simulink model "serial3_sm_ROS"  (R2022a)
settings: Solver=VariableStepAuto  StartTime=0.0  StopTime=inf  RelTol=1e-3
libraries: robotlib x8
settings Model: Creator=johnc  LastModifiedBy=johnc
settings SolverCC: AlgebraicLoopSolver=TrustRegion
settings DebuggingCC: UnconnectedInputMsg=warning  UnconnectedOutputMsg=warning  UnconnectedLineMsg=warning  SFMachineParentedDataDiag=warning

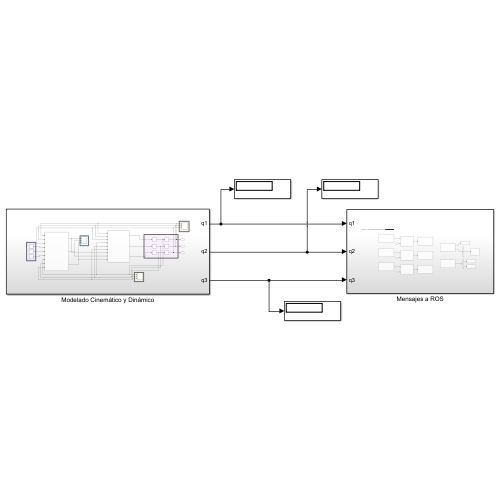
[thumbnail: Simulink's stored preview of the top-level diagram]
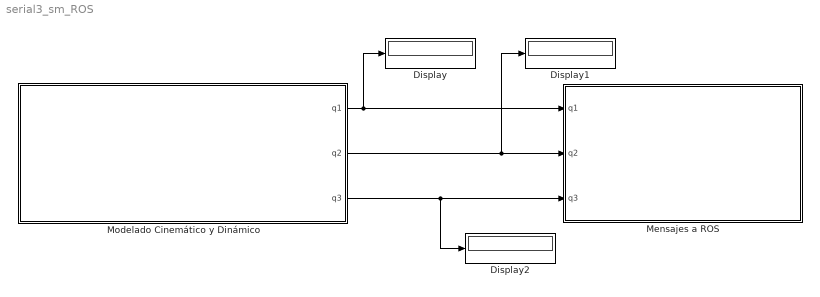
== system serial3_sm_ROS ==
  Display : Display
  Display1 : Display
  Display2 : Display
  Mensajes a ROS : Subsystem
  Modelado Cinemático y Dinámico : Subsystem
  wires:
  Modelado Cinemático y Dinámico/1(q1) -> Display/1, Mensajes a ROS/1(q1)
  Modelado Cinemático y Dinámico/2(q2) -> Display1/1, Mensajes a ROS/2(q2)
  Modelado Cinemático y Dinámico/3(q3) -> Display2/1, Mensajes a ROS/3(q3)

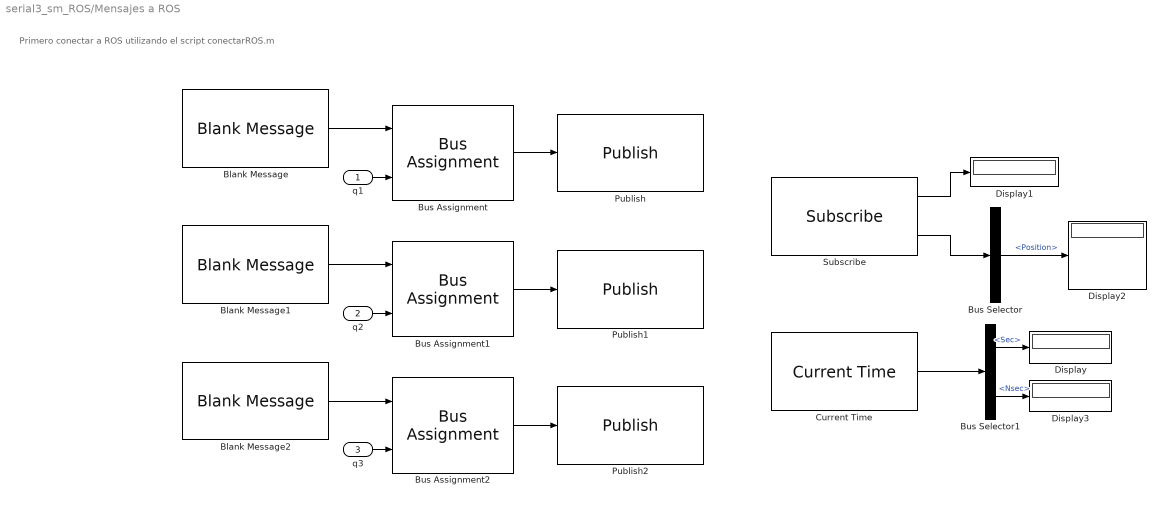
== system serial3_sm_ROS/Mensajes a ROS ==
  note: Primero conectar a ROS utilizando el script conectarROS.m
  q1 : Inport
  q2 : Inport  Port=2
  q3 : Inport  Port=3
  Blank Message : robotlib/Blank Message  messageClass=Message  entityType=std_msgs/Float64  messageType=std_msgs/Float64  SampleTime=inf  legacyBusStruct=off
  Blank Message1 : robotlib/Blank Message  messageClass=Message  entityType=std_msgs/Float64  messageType=std_msgs/Float64  SampleTime=inf  legacyBusStruct=off
  Blank Message2 : robotlib/Blank Message  messageClass=Message  entityType=std_msgs/Float64  messageType=std_msgs/Float64  SampleTime=inf  legacyBusStruct=off
  Bus Assignment : BusAssignment  AssignedSignals=Data
  Bus Assignment1 : BusAssignment  AssignedSignals=Data
  Bus Assignment2 : BusAssignment  AssignedSignals=Data
  Bus Selector : BusSelector  OutputSignals=Position
  Bus Selector1 : BusSelector  OutputSignals=Sec,Nsec
  Current Time : robotlib/Current Time  OutputFormat=bus  SampleTime=-1  ModelName=serial3_modeloROS
      settings: SourceProductBaseCode=RR
  Display{,1..3} (4 alike) : Display
  Publish : robotlib/Publish  topicSource=Select from ROS network  topic=/serial3/joint_e1_position_controller/command  messageType=std_msgs/Float64  legacyBusStruct=off  messageQueueLength=1
  Publish1 : robotlib/Publish  topicSource=Select from ROS network  topic=/serial3/joint_e2_position_controller/command  messageType=std_msgs/Float64  legacyBusStruct=off  messageQueueLength=1
  Publish2 : robotlib/Publish  topicSource=Select from ROS network  topic=/serial3/joint_e3_position_controller/command  messageType=std_msgs/Float64  legacyBusStruct=off  messageQueueLength=1
  Subscribe : robotlib/Subscribe  topicSource=Select from ROS network  topic=/serial3/joint_states  messageType=sensor_msgs/JointState  SampleTime=-1  legacyBusStruct=off  messageQueueLength=1
  wires:
  Blank Message2/1 -> Bus Assignment2/1
  Blank Message/1 -> Bus Assignment/1
  Bus Assignment2/1 -> Publish2/1
  q1/1 -> Bus Assignment/2
  Bus Assignment/1 -> Publish/1
  Blank Message1/1 -> Bus Assignment1/1
  Bus Assignment1/1 -> Publish1/1
  q3/1 -> Bus Assignment2/2
  q2/1 -> Bus Assignment1/2
  Subscribe/2 -> Bus Selector/1
  Subscribe/1 -> Display1/1
  Bus Selector/1 -> Display2/1  "<Position>"
  Current Time/1 -> Bus Selector1/1
  Bus Selector1/1 -> Display/1  "<Sec>"
  Bus Selector1/2 -> Display3/1  "<Nsec>"

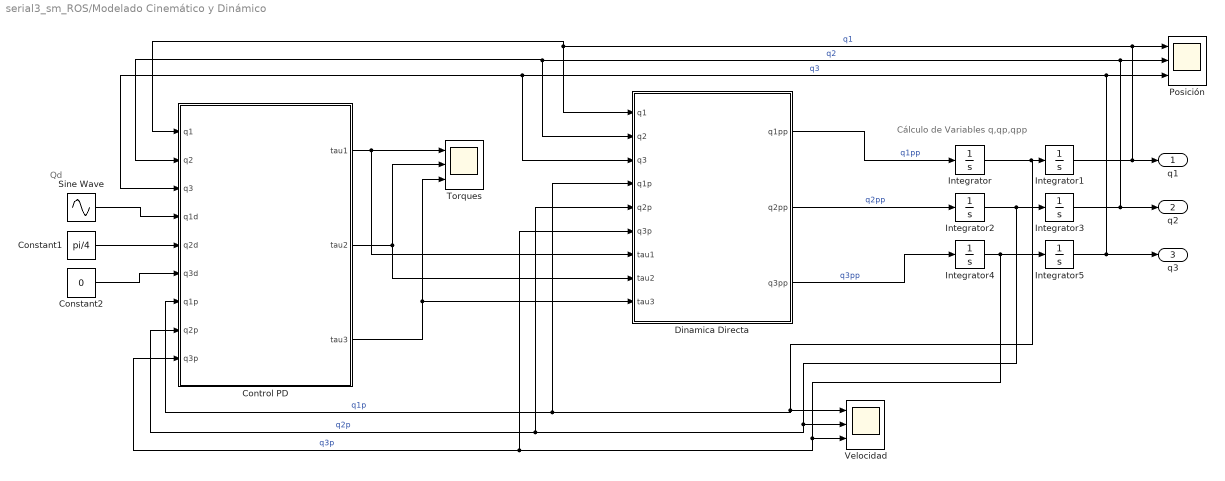
== system serial3_sm_ROS/Modelado Cinemático y Dinámico ==
  note: Qd
  note: Cálculo de Variables q,qp,qpp
  Constant1 : Constant  Value=pi/4
  Constant2 : Constant  Value=0
  Control PD : MATLAB Function  TreatAsAtomicUnit=on
  Dinamica Directa : MATLAB Function  TreatAsAtomicUnit=on
  Integrator{,1..5} (6 alike) : Integrator
  Posición : Scope  NumInputPorts=3
  Sine Wave : Sin  SampleTime=0
  Torques : Scope  NumInputPorts=3
  Velocidad : Scope  NumInputPorts=3
  q1 : Outport  VectorParamsAs1DForOutWhenUnconnected=off
  q2 : Outport  Port=2  VectorParamsAs1DForOutWhenUnconnected=off
  q3 : Outport  Port=3  VectorParamsAs1DForOutWhenUnconnected=off
  wires:
  Integrator2/1 -> Integrator3/1, Dinamica Directa/5(q2p), Control PD/8(q2p), Velocidad/2  "q2p"
  Control PD/1(tau1) -> Dinamica Directa/7(tau1), Torques/1
  Constant2/1 -> Control PD/6(q3d)
  Integrator3/1 -> Posición/2, Control PD/2(q2), Dinamica Directa/2(q2), q2/1  "q2"
  Integrator/1 -> Dinamica Directa/4(q1p), Control PD/7(q1p), Velocidad/1, Integrator1/1  "q1p"
  Dinamica Directa/2(q2pp) -> Integrator2/1  "q2pp"
  Control PD/3(tau3) -> Torques/3, Dinamica Directa/9(tau3)
  Dinamica Directa/1(q1pp) -> Integrator/1  "q1pp"
  Dinamica Directa/3(q3pp) -> Integrator4/1  "q3pp"
  Integrator1/1 -> q1/1, Control PD/1(q1), Dinamica Directa/1(q1), Posición/1  "q1"
  Control PD/2(tau2) -> Torques/2, Dinamica Directa/8(tau2)
  Integrator4/1 -> Dinamica Directa/6(q3p), Control PD/9(q3p), Velocidad/3, Integrator5/1  "q3p"
  Constant1/1 -> Control PD/5(q2d)
  Integrator5/1 -> q3/1, Dinamica Directa/3(q3), Control PD/3(q3), Posición/3  "q3"
  Sine Wave/1 -> Control PD/4(q1d)

== matlab function serial3_sm_ROS/Modelado Cinemático y Dinámico/Dinamica Directa ==
  data: q1 input; q1pp output; q2 input; q3 input; q1p input; q2p input; q3p input; tau1 input; tau2 input; tau3 input; q2pp output; q3pp output
function [q1pp,q2pp,q3pp] = din_directa(q1,q2,q3,q1p,q2p,q3p,tau1,tau2,tau3)

M =[ (5589*cos(q3))/20000000 - (833252400176387296733*cos(2*q2))/5764607523034234880000000 - (12569150243223845732103*cos(2*q2 + 2*q3))/92233720368547758080000000 - (5589*cos(2*q2 + q3))/20000000 + 51717330115768924042331/92233720368547758080000000,                                    0,                                     0;
                                                                                                                                                                                                                                                   0, 5676674199877871/4611686018427387904,  5351169871482219/9223372036854775808;
                                                                                                                                                                                                                                                 0, 5351169871482219/9223372036854775808, 5547397111566305/18446744073709551616];
 
G =[0;-(42678181724791417*sin(q2+q3))/1801439850948198400-(3884277835938411*sin(q2))/28147497671065600;-(6828509075966627*sin(q2 + q3))/288230376151711744];
 
 
C = [q1p*((833252400176387296733*q2p*sin(2*q2))/2882303761517117440000000 + (12569150243223845732103*q2p*sin(2*q2 + 2*q3))/46116860184273879040000000 + (12569150243223845732103*q3p*sin(2*q2 + 2*q3))/46116860184273879040000000 - (5589*q3p*sin(q3))/20000000 + (5589*q2p*sin(2*q2 + q3))/10000000 + (5589*q3p*sin(2*q2 + q3))/20000000);
                                                                                                                                                     -(q1p^2*((5589*sin(2*q2 + q3))/10000000 + (833252400176387296733*sin(2*q2))/2882303761517117440000000 + (12569150243223845732103*sin(2*q2 + 2*q3))/46116860184273879040000000))/2;
                                                                                                                                                                                         -(q1p^2*((5589*sin(2*q2 + q3))/20000000 + (12569150243223845732103*sin(2*q2 + 2*q3))/46116860184273879040000000 - (5589*sin(q3))/20000000))/2];
Fm1=0.123;
F=[Fm1*q1p;Fm1*q2p;Fm1*q3p];    %Friccion de las juntas - Funcion disipativa

Tau=[tau1;tau2;tau3];
qpp=(inv(M))*(Tau-C-G-F);
q1pp=qpp(1);
q2pp=qpp(2);
q3pp=qpp(3);

== matlab function serial3_sm_ROS/Modelado Cinemático y Dinámico/Control PD ==
  data: q1 input; tau1 output; q2 input; q3 input; q1d input; q2d input; q3d input; q1p input; q2p input; q3p input; tau2 output; tau3 output
function [tau1,tau2,tau3] = controlpd(q1,q2,q3,q1d,q2d,q3d,q1p,q2p,q3p)

kp=1;
kv=0.02;

Kp=[kp 0 0;0 kp 0;0 0 kp];
Kv=[kv 0 0;0 kv 0;0 0 kv];

qe=[q1d-q1;q2d-q2;q3d-q3];

qp=[q1;q2;q3];

G =[0;-(42678181724791417*sin(q2+q3))/1801439850948198400-(3884277835938411*sin(q2))/28147497671065600;-(6828509075966627*sin(q2 + q3))/288230376151711744];
 
Tau=Kp*qe-Kv*qp+G;
tau1=Tau(1);
tau2=Tau(2);
tau3=Tau(3);
